simulink model "Main"  (R2020a)
settings: Solver=VariableStepAuto  StartTime=0.0  StopTime=5  RelTol=1e-3
libraries: audiosources x1, simulink x1, dspvision x1
settings Model: Creator=Emil  LastModifiedBy=Emil

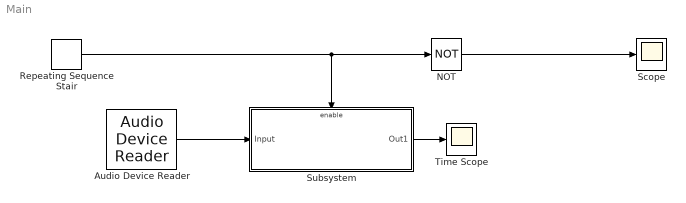
== system Main ==
  Audio Device Reader : audiosources/Audio Device Reader  Driver=DirectSound  Device=Default  SampleRate=44100  NumChannels=1  SamplesPerFrame=1024  BitDepth=16-bit integer  NumBuffers=10  DefaultInputChannelMapping=on  InputChannelMapping=1:2  OutputNumOverrunSamples=off  OutputDataType=double  DriverIdx=1  DeviceWarnFlag=''
      settings: SourceProductBaseCode=AU
  NOT : Logic  Operator=NOT  IconShape=distinctive  AllPortsSameDT=off  OutDataTypeStr=boolean
  Repeating Sequence Stair : simulink/Sources/Repeating Sequence Stair  OutValues=[1 1 1 1 1 0 0 0 0 0].'  tsamp=0.5  OutMin=[]  OutMax=[]  OutDataTypeStr=double  OutputDataTypeScalingMode=double  OutDataType=fixdt(0,8)  ConRadixGroup=Best Precision: Vector-wise  OutScaling=2^-12
  Scope : Scope
  Subsystem : Subsystem
  Time Scope : Scope
  wires:
  Subsystem/1(Out1) -> Time Scope/1
  Repeating Sequence Stair/1 -> NOT/1, Subsystem/Enable
  Audio Device Reader/1 -> Subsystem/1(Input)
  NOT/1 -> Scope/1

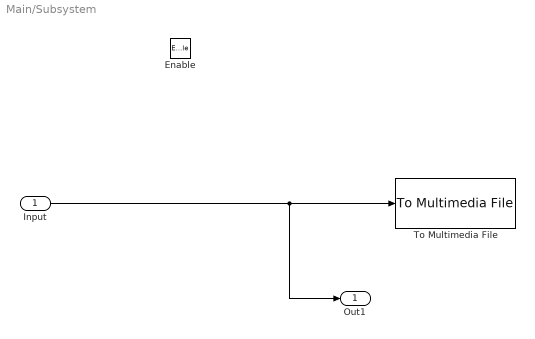
== system Main/Subsystem ==
  Input : Inport
  Enable : EnablePort
  To Multimedia File : dspvision/To Multimedia File  outputFilename=Test.wav  streamSelection=Audio only  videoCompressor=None (uncompressed)  audioCompressor=None (uncompressed)  imagePorts=Separate color signals  fileType=WAV  audioDatatype=16-bit integer  fourcc=RGB  videoQuality=75  mj2000CompFactor=10
  Out1 : Outport
  wires:
  Input/1 -> Out1/1, To Multimedia File/1
